simulink model "shifter_blocks"  (R2022b)
settings: Solver=FixedStepDiscrete  StartTime=0.0  StopTime=30  FixedStep=0.05  RelTol=1e-3  EnableMultiTasking=on
PreLoadFcn:
  | % Input data
  | load shifter_data;
settings Model: Creator=jrivitus  LastModifiedBy=bensweet
settings SolverCC: AlgebraicLoopSolver=TrustRegion
settings DataIOCC: ExternalInput=[t, upThreshold, vehicleSpeed, downThreshold]  LimitDataPoints=on  LoadExternalInput=on  SaveFormat=Array  ReturnWorkspaceOutputs=off
settings OptimizationCC: ExpressionDepthLimit=2147483647  LifeSpan=inf
settings DebuggingCC: UnconnectedInputMsg=warning  UnconnectedOutputMsg=warning  UnconnectedLineMsg=warning  PregeneratedLibrarySubsystemCodeDiagnostic=none  SFMachineParentedDataDiag=warning
settings HardwareCC: ProdBitPerPointer=32  ProdBitPerSizeT=32  ProdBitPerPtrDiffT=32  ProdLargestAtomicFloat=None  ProdIntDivRoundTo=Undefined  ProdEndianess=Unspecified  ProdWordSize=32  ProdHWDeviceType=32-bit Generic
settings ModelReferenceCC: EnableRefExpFcnMdlSchedulingChecks=on  PropagateSignalLabelsOutOfModel=off
settings SFSimCC: SimUseLocalCustomCode=off
settings RTWCC: RTWUseLocalCustomCode=off  DLArmComputeVersion=19.05
settings CodeAppCC: StateflowObjectComments=on
settings GRTTargetCC: TargetLangStandard=C89/C90 (ANSI)  CombineOutputUpdateFcns=off  GRTInterface=on
settings ConfigComp: CovMetricSettings=dw  CovSaveCumulativeToWorkspaceVar=on  CovSaveSingleToWorkspaceVar=on  CovExternalEMLEnable=off  CovSFcnEnable=off

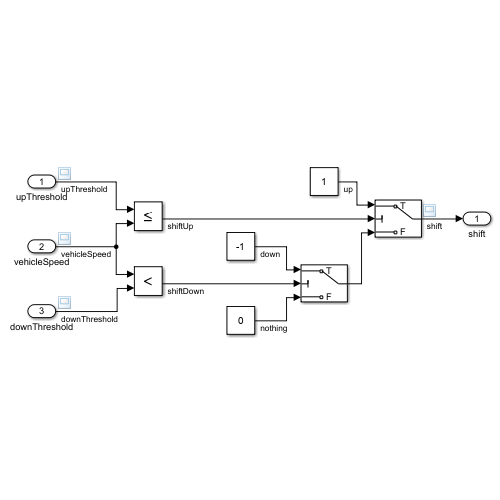
[thumbnail: Simulink's stored preview of the top-level diagram]
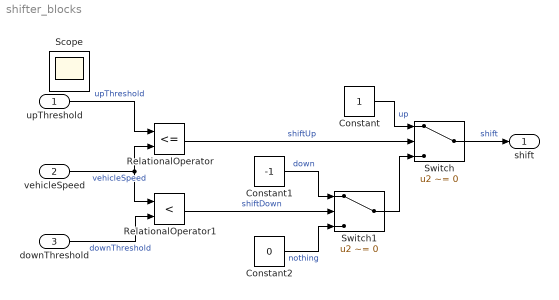
== system shifter_blocks ==
  upThreshold : Inport  OutDataTypeStr=double
  vehicleSpeed : Inport  Port=2  OutDataTypeStr=double
  downThreshold : Inport  Port=3  OutDataTypeStr=double
  Constant : Constant
  Constant1 : Constant  Value=-1
  Constant2 : Constant  Value=0
  RelationalOperator : RelationalOperator  Operator=<=  OutDataTypeStr=boolean  InputSameDT=off
  RelationalOperator1 : RelationalOperator  Operator=<  OutDataTypeStr=boolean  InputSameDT=off
  Switch : Switch  Criteria=u2 ~= 0  SaturateOnIntegerOverflow=off  InputSameDT=off
  Switch1 : Switch  Criteria=u2 ~= 0  SaturateOnIntegerOverflow=off  InputSameDT=off
  shift : Outport  VectorParamsAs1DForOutWhenUnconnected=off
  Scope : Scope
  wires:
  RelationalOperator/1 -> Switch/2  "shiftUp"
  upThreshold/1 -> RelationalOperator/1  "upThreshold"
  vehicleSpeed/1 -> RelationalOperator/2, RelationalOperator1/1  "vehicleSpeed"
  RelationalOperator1/1 -> Switch1/2  "shiftDown"
  downThreshold/1 -> RelationalOperator1/2  "downThreshold"
  Constant/1 -> Switch/1  "up"
  Constant1/1 -> Switch1/1  "down"
  Constant2/1 -> Switch1/3  "nothing"
  Switch1/1 -> Switch/3
  Switch/1 -> shift/1  "shift"
